simulink model "Lab1_OBS"  (R2023b)
settings: Solver=FixedStepAuto  StartTime=0.0  StopTime=5  FixedStep=.01  RelTol=1e-3
undefined symbols (not defined in the file or in its folder): A, B, C, K, L
settings Model: Creator=Connor Emmons  LastModifiedBy=Connor Emmons

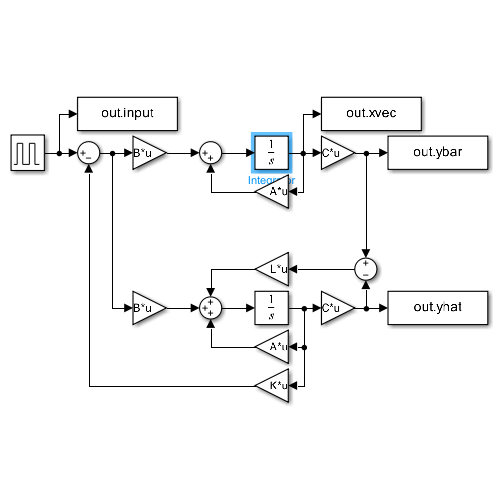
[thumbnail: Simulink's stored preview of the top-level diagram]
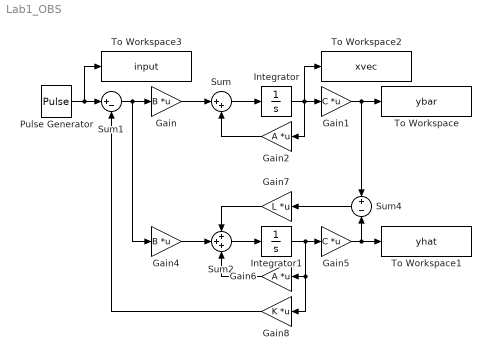
== system Lab1_OBS ==
  Gain : Gain  Gain=B  Multiplication=Matrix(K*u)
  Gain1 : Gain  Gain=C  Multiplication=Matrix(K*u)
  Gain2 : Gain  Gain=A  Multiplication=Matrix(K*u)
  Gain4 : Gain  Gain=B  Multiplication=Matrix(K*u)
  Gain5 : Gain  Gain=C  Multiplication=Matrix(K*u)
  Gain6 : Gain  Gain=A  Multiplication=Matrix(K*u)
  Gain7 : Gain  Gain=L  Multiplication=Matrix(K*u)
  Gain8 : Gain  Gain=K  Multiplication=Matrix(K*u)
  Integrator : Integrator
  Integrator1 : Integrator  InitialCondition=[0.2; 0.2]
  Pulse Generator : DiscretePulseGenerator  PulseType=Time based  Period=10  PulseWidth=5
  Sum : Sum  Inputs=|++
  Sum1 : Sum  Inputs=|+-
  Sum2 : Sum  Inputs=+++
  Sum4 : Sum  Inputs=+-
  To Workspace : ToWorkspace  VariableName=ybar  SampleTime=-1
  To Workspace1 : ToWorkspace  VariableName=yhat  SampleTime=-1
  To Workspace2 : ToWorkspace  VariableName=xvec  SampleTime=-1
  To Workspace3 : ToWorkspace  VariableName=input  SampleTime=-1
  wires:
  Gain/1 -> Sum/1
  Sum/1 -> Integrator/1
  Integrator/1 -> To Workspace2/1, Gain1/1, Gain2/1
  Gain2/1 -> Sum/2
  Sum1/1 -> Gain4/1, Gain/1
  Pulse Generator/1 -> To Workspace3/1, Sum1/1
  Gain1/1 -> Sum4/1, To Workspace/1
  Integrator1/1 -> Gain8/1, Gain6/1, Gain5/1
  Sum2/1 -> Integrator1/1
  Gain5/1 -> Sum4/2, To Workspace1/1
  Sum4/1 -> Gain7/1
  Gain4/1 -> Sum2/2
  Gain6/1 -> Sum2/3
  Gain7/1 -> Sum2/1
  Gain8/1 -> Sum1/2
